simulink model "dsds"  (R2023b)
settings: Solver=VariableStepAuto  StartTime=0.0  StopTime=100.0  RelTol=1e-3
values from neighbouring files (symbols this model uses):
  f = 0.2    [aaa.m]    (also in matlab.mat)
  J = 1    [aaa.m]    (also in matlab.mat)
  Ka = 0.05    [aaa.m]    (also in matlab.mat)
  Kb = 0.5    [aaa.m]    (also in matlab.mat)
  Kt = 1    [aaa.m]    (also in matlab.mat)
libraries: simulink x1
settings Model: Creator=nilfam  LastModifiedBy=nilfam

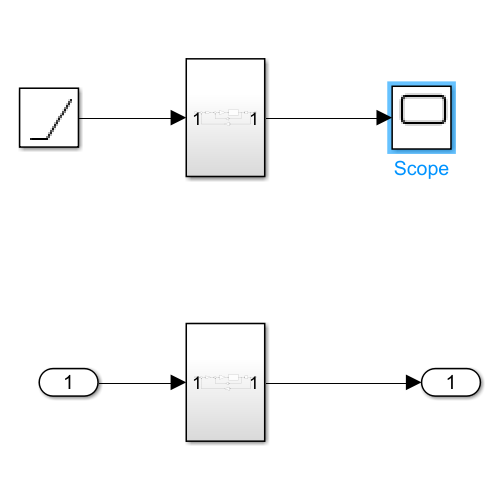
[thumbnail: Simulink's stored preview of the top-level diagram]
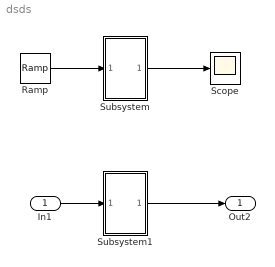
== system dsds ==
  In1 : Inport
  Ramp : simulink/Sources/Ramp  slope=1  start=0  InitialOutput=0
  Scope : Scope
  Subsystem : Subsystem
  Subsystem1 : Subsystem
  Out2 : Outport
  wires:
  Ramp/1 -> Subsystem/1(In1)
  Subsystem/1(Out1) -> Scope/1
  In1/1 -> Subsystem1/1(In1)
  Subsystem1/1(Out1) -> Out2/1

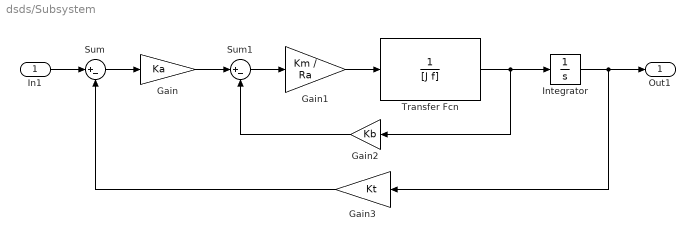
== system dsds/Subsystem ==
  In1 : Inport
  Gain : Gain  Gain=Ka
  Gain1 : Gain  Gain=Km / Ra
  Gain2 : Gain  Gain=Kb
  Gain3 : Gain  Gain=Kt
  Integrator : Integrator
  Sum : Sum  Inputs=|+-
  Sum1 : Sum  Inputs=|+-
  Transfer Fcn : TransferFcn  Denominator=[J f]
  Out1 : Outport
  wires:
  Transfer Fcn/1 -> Gain2/1, Integrator/1
  Integrator/1 -> Out1/1, Gain3/1
  Sum/1 -> Gain/1
  Gain3/1 -> Sum/2
  Gain/1 -> Sum1/1
  Sum1/1 -> Gain1/1
  Gain1/1 -> Transfer Fcn/1
  Gain2/1 -> Sum1/2
  In1/1 -> Sum/1

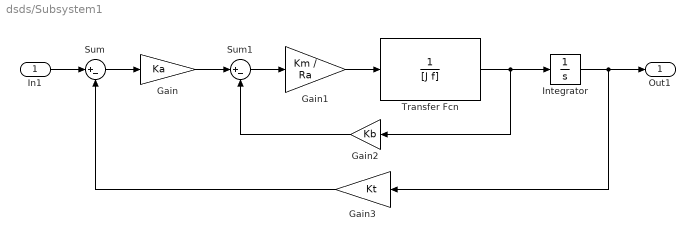
== system dsds/Subsystem1 ==
  In1 : Inport
  Gain : Gain  Gain=Ka
  Gain1 : Gain  Gain=Km / Ra
  Gain2 : Gain  Gain=Kb
  Gain3 : Gain  Gain=Kt
  Integrator : Integrator
  Sum : Sum  Inputs=|+-
  Sum1 : Sum  Inputs=|+-
  Transfer Fcn : TransferFcn  Denominator=[J f]
  Out1 : Outport
  wires:
  Transfer Fcn/1 -> Gain2/1, Integrator/1
  Integrator/1 -> Out1/1, Gain3/1
  Sum/1 -> Gain/1
  Gain3/1 -> Sum/2
  Gain/1 -> Sum1/1
  Sum1/1 -> Gain1/1
  Gain1/1 -> Transfer Fcn/1
  Gain2/1 -> Sum1/2
  In1/1 -> Sum/1
